simulink model "whipple_bicycle"  (R2022b)
settings: Solver=VariableStepAuto  StartTime=0.0  StopTime=10.0  RelTol=1e-3
InitFcn:
  | whipple_bicycle_params;
values from neighbouring files (symbols this model uses):
  params = [I_bx I_bxz I_by I_bz I_fx I_fy I_fz I_hx I_hxz I_hy I_hz I_rx I_ry I_rz b d e f g h m_b m_f m_h m_r p r_f r_r varepsilon].'    [whipple_bicycle_params.m]
  x0 = [ ... (first row only)    [whipple_bicycle_params.m]
settings Model: Creator=marti  LastModifiedBy=marti

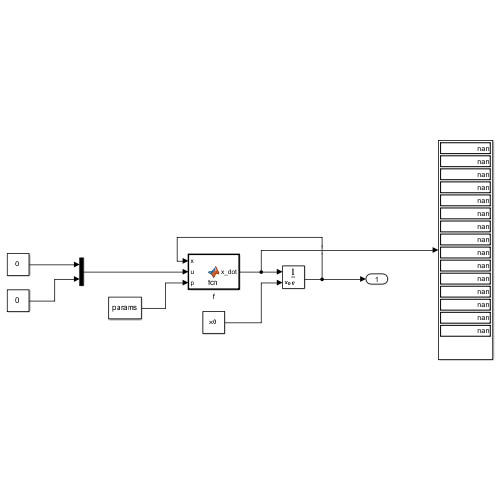
[thumbnail: Simulink's stored preview of the top-level diagram]
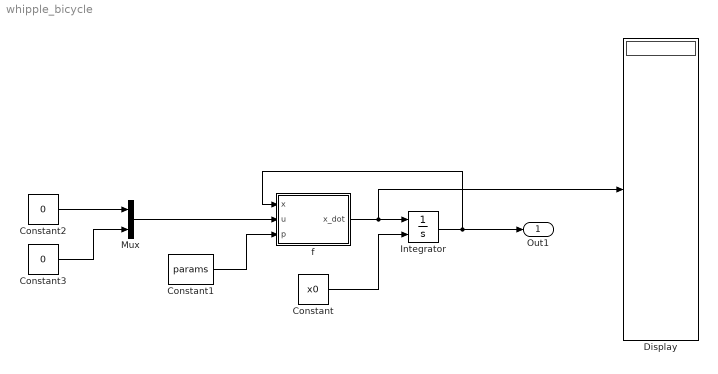
== system whipple_bicycle ==
  Constant : Constant  Value=x0
  Constant1 : Constant  Value=params
  Constant2 : Constant  Value=0
  Constant3 : Constant  Value=0
  Display : Display
  Integrator : Integrator  InitialConditionSource=external
  Mux : Mux  Inputs=2
  f : MATLAB Function  TreatAsAtomicUnit=on
  Out1 : Outport
  wires:
  f/1(x_dot) -> Display/1, Integrator/1
  Constant/1 -> Integrator/2
  Constant1/1 -> f/3(p)
  Integrator/1 -> Out1/1, f/1(x)
  Mux/1 -> f/2(u)
  Constant2/1 -> Mux/1
  Constant3/1 -> Mux/2

== matlab function whipple_bicycle/f ==
  data: x input; u input; p input; x_dot output
function x_dot = fcn(x,u,p)
x_dot = whippleBicycle(x,u,p);
